simulink model "gantrycrane_animation"  (Simulink 7.9)
settings: Solver=ode45  StartTime=0.0  StopTime=10000  RelTol=1e-3
undefined symbols (not defined in the file or in its folder): drawGantryCrane
libraries: simulink x3
settings Model: Creator=nedward  LastModifiedBy=timmclain
settings DebuggingCC: FcnCallInpInsideContextMsg=Use local settings
settings GRTTargetCC: CombineOutputUpdateFcns=off  GRTInterface=on

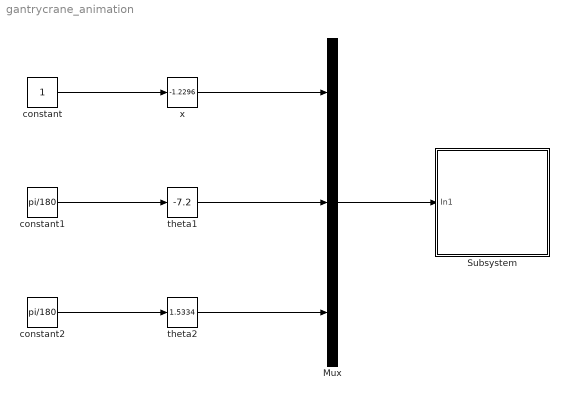
== system gantrycrane_animation ==
  Mux : Mux  Inputs=3
  Subsystem : Subsystem
      mask init:
      | bar = 20;
      | crane = [5 3];
      | L1 = 5;
      | R1 = 1;
      | L2 = 10;
      | R2 = 0.5;
      mask Display: image(imread('tv.jpg'))
  constant : Constant
  constant1 : Constant  Value=pi/180
  constant2 : Constant  Value=pi/180
  theta1 : simulink/Math Operations/Slider Gain  low=-90  gain=-7.2  high=90
  theta2 : simulink/Math Operations/Slider Gain  low=-90  gain=1.5334  high=90
  x : simulink/Math Operations/Slider Gain  low=-10  gain=-1.2296  high=10
  wires:
  constant/1 -> x/1
  x/1 -> Mux/1
  constant1/1 -> theta1/1
  theta1/1 -> Mux/2
  constant2/1 -> theta2/1
  theta2/1 -> Mux/3
  Mux/1 -> Subsystem/1(In1)

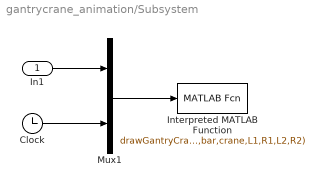
== system gantrycrane_animation/Subsystem ==
  In1 : Inport
  Clock : Clock
  Interpreted MATLAB Function : MATLABFcn  MATLABFcn=drawGantryCrane(u,bar,crane,L1,R1,L2,R2)  OutputDimensions=0  SampleTime=0.1
  Mux1 : Mux  Inputs=2
  wires:
  Clock/1 -> Mux1/2
  Mux1/1 -> Interpreted MATLAB Function/1
  In1/1 -> Mux1/1
